simulink model "RASCAL72_cl"  (R2017b)
settings: Solver=FixedStepDiscrete  StartTime=0.0  StopTime=100  RelTol=1e-3  EnableMultiTasking=on
values from neighbouring files (symbols this model uses):
  CD0 = 0.0164    [Final_Project_START.m]
  CDa_200 = [0.53 0.53 0.53 0.53 0.53 0.53 0.53 0.53 0.53 0.53 0.53 0.53 ... (25 elements, 5x5)]    [C1o_200.mat]    (also in CDa_200.mat; CLadot_200.mat; CLde.mat; CLo_200.mat)
  CDde_200 = [0 0 0 0 0 0 0 0 0 0 0 0 ... (25 elements, 5x5)]    [C1o_200.mat]    (also in CDde_200.mat; CLadot_200.mat; CLde.mat; CLo_200.mat)
  CDq_200 = [0 0 0 0 0 0 0 0 0 0 0 0 ... (25 elements, 5x5)]    [C1o_200.mat]    (also in CDq_200.mat; CLadot_200.mat; CLde.mat; CLo_200.mat)
  CL0 = 0.21    [Final_Project_START.m]
  Cl0 = 0    [Final_Project_START.m]
  CLa_200 = [5.326215664 5.440234265 5.741037107 5.849899088 5.539928921 5.331372284 5.445390885 5.746766685 5.849899088 5.539355963 5.335955946 5.449401589 ... (25 elements, 5x5)]    [C1o_200.mat]    (also in CLa_200.mat; CLadot_200.mat; CLde.mat; CLo_200.mat)
  ClB_200 = [-0.052500123 -0.052614714 -0.052614714 -0.05294703 -0.053136106 -0.052523041 -0.052649092 -0.052666281 -0.053015785 -0.05322205 -0.052545959 -0.0525345 ... (25 elements, 5x5)]    [C1B_200.mat]    (also in C1o_200.mat; CLadot_200.mat; Cma_200.mat; Cmadot_200.mat)
  Clda_200 = [0.03678389 0.037299552 0.037299552 0.036726595 0.035580679 0.03678389 0.037299552 0.037299552 0.036726595 0.035580679 0.03678389 0.037299552 ... (25 elements, 5x5)]    [C1da_200.mat]    (also in C1o_200.mat = [0.000642 0.000651 0.000651 0.000641 0.000621 0.000642 0.000; CLadot_200.mat = [0.000642 0.000651 0.000651 0.000641 0.000621 0.000642 0.000; Cma_200.mat = [0.000642 0.000651 0.000651 0.000641 0.000621 0.000642 0.000; Cmadot_200.mat = [0.000642 0.000651 0.000651 0.000641 0.000621 0.000642 0.000)
  CLde_200 = [0.001609 0.00164 0.001639 0.001604 0.001542 0.001609 0.00164 0.001639 0.001604 0.001542 0.001609 0.00164 ... (25 elements, 5x5)]    [C1o_200.mat]    (also in CLadot_200.mat; CLde.mat; CLde_200.mat = [0.092188909 0.093965078 0.093907783 0.09190243 0.088350092 ; CLo_200.mat)
  Cldr_200 = [-5.72958e-05 0 5.72958e-05 0.000114592 0.000171887 -5.72958e-05 0 5.72958e-05 0.000114592 0.000171887 -5.72958e-05 0 ... (25 elements, 5x5)]    [C1dr_200.mat]    (also in C1o_200.mat = [-1e-06 0 1e-06 2e-06 3e-06 -1e-06 0 1e-06 2e-06 3e-06 -1e-0; CLadot_200.mat = [-1e-06 0 1e-06 2e-06 3e-06 -1e-06 0 1e-06 2e-06 3e-06 -1e-0; Cma_200.mat = [-1e-06 0 1e-06 2e-06 3e-06 -1e-06 0 1e-06 2e-06 3e-06 -1e-0; Cmadot_200.mat = [-1e-06 0 1e-06 2e-06 3e-06 -1e-06 0 1e-06 2e-06 3e-06 -1e-0)
  Clp_200 = [-0.448740545 -0.460829955 -0.490337281 -0.496124155 -0.462205053 -0.448740545 -0.460772659 -0.490279985 -0.496009563 -0.461861279 -0.448797841 -0.460829955 ... (25 elements, 5x5)]    [C1o_200.mat]    (also in C1p_200.mat; CLadot_200.mat; Cma_200.mat; Cmadot_200.mat)
  CLq_200 = [9.310564171 9.310564171 9.310564171 9.310564171 9.310564171 9.344941639 9.344941639 9.344941639 9.344941639 9.344941639 9.373589528 9.373589528 ... (25 elements, 5x5)]    [C1o_200.mat]    (also in CLadot_200.mat; CLde.mat; CLo_200.mat; CLq_200.mat)
  Clr_200 = [-0.074885584 0.016254813 0.110122488 0.213369483 0.308595068 -0.07494288 0.016260542 0.11023708 0.21354137 0.308824252 -0.075000175 0.016272001 ... (25 elements, 5x5)]    [C1o_200.mat]    (also in C1r_200.mat; CLadot_200.mat; CLde.mat; CLo_200.mat)
  Cm0 = 0    [Final_Project_START.m]
  Cma_200 = [-1.61689 -1.94061 -2.12224 -2.54508 -2.95302 -1.61918 -1.94978 -2.1314 -2.55367 -2.96506 -1.62319 -1.9578 ... (25 elements, 5x5)]    [C1o_200.mat]    (also in CLadot_200.mat; CLde.mat; CLo_200.mat; CLq_200.mat)
  Cmde_200 = [-0.002239 -0.002272 -0.00227 -0.00223 -0.002161 -0.002239 -0.002272 -0.00227 -0.00223 -0.002161 -0.002239 -0.002272 ... (25 elements, 5x5)]    [C1o_200.mat]    (also in CLadot_200.mat; CLde.mat; CLo_200.mat; CLq_200.mat)
  Cmq_200 = [-17.06841272 -17.06841272 -17.06841272 -17.06841272 -17.06841272 -17.17154512 -17.17154512 -17.17154512 -17.17154512 -17.17154512 -17.25175921 -17.25175921 ... (25 elements, 5x5)]    [C1o_200.mat]    (also in CLadot_200.mat; CLde.mat; CLo_200.mat; CLq_200.mat)
  Cn0 = 0    [Final_Project_START.m]
  CnB_200 = [0.029759428 0.029759428 0.029759428 0.029759428 0.029759428 0.028264008 0.028264008 0.028264008 0.028264008 0.028264008 0.027209766 0.027209766 ... (25 elements, 5x5)]    [C1o_200.mat]    (also in CLadot_200.mat; CLde.mat; CLo_200.mat; CLq_200.mat)
  Cnda_200 = [-4.5e-05 -2.9e-05 -1.1e-05 6e-06 2.2e-05 -4.5e-05 -2.9e-05 -1.1e-05 6e-06 2.2e-05 -4.5e-05 -2.9e-05 ... (25 elements, 5x5)]    [C1o_200.mat]    (also in CLadot_200.mat; CLde.mat; CLo_200.mat; CLq_200.mat)
  Cndr_200 = [0.000151 0.000159 0.000163 0.000164 0.00016 0.000151 0.000159 0.000163 0.000164 0.00016 0.000151 0.000159 ... (25 elements, 5x5)]    [C1o_200.mat]    (also in CLadot_200.mat; CLde.mat; CLo_200.mat; CLq_200.mat)
  Cnp_200 = [0.038193 0.000534 -0.03759 -0.07993 -0.12032 0.039712 0.000373 -0.03967 -0.08394 -0.12594 0.040583 0.00028 ... (25 elements, 5x5)]    [C1o_200.mat]    (also in CLadot_200.mat; CLde.mat; CLo_200.mat; CLq_200.mat)
  Cnr_200 = [-0.040473739 -0.043229666 -0.042771299 -0.038405361 -0.030859507 -0.040015372 -0.042908809 -0.042244178 -0.037247986 -0.028751022 -0.039728894 -0.042702544 ... (25 elements, 5x5)]    [C1o_200.mat]    (also in CLadot_200.mat; CLde.mat; CLo_200.mat; CLq_200.mat)
  CY0 = 0    [Final_Project_START.m]
  CYB_200 = [-0.504374747 -0.504374747 -0.504374747 -0.504374747 -0.504374747 -0.504374747 -0.504374747 -0.504374747 -0.504374747 -0.504374747 -0.504432043 -0.50432043 ... (25 elements, 5x5)]    [C1o_200.mat]    (also in CLadot_200.mat; CLde.mat; CLo_200.mat; CLq_200.mat)
  CYda_200 = [4e-06 2.7e-05 5e-05 7.1e-05 9.1e-05 4e-06 2.7e-05 5e-05 7.1e-05 9.1e-05 4e-06 2.7e-05 ... (25 elements, 5x5)]    [C1o_200.mat]    (also in CLadot_200.mat; CLde.mat; CLo_200.mat; CLq_200.mat)
  CYdr_200 = [-0.000731 -0.000766 -0.000782 -0.00078 -0.000759 -0.000731 -0.000766 -0.000782 -0.00078 -0.000759 -0.000731 -0.000766 ... (25 elements, 5x5)]    [C1o_200.mat]    (also in CLadot_200.mat; CLde.mat; CLo_200.mat; CLq_200.mat)
  CYp_200 = [-0.030521462 -0.058498991 -0.087204176 -0.119576292 -0.14919821 -0.029782346 -0.058613582 -0.088178205 -0.121581644 -0.152005703 -0.029358357 -0.058670878 ... (25 elements, 5x5)]    [C1o_200.mat]    (also in CLadot_200.mat; CLde.mat; CLo_200.mat; CLq_200.mat)
  CYr_200 = [0.026877 0.03248 0.035656 0.0363 0.03441 0.026877 0.03248 0.035656 0.0363 0.03441 0.026877 0.03248 ... (25 elements, 5x5)]    [C1o_200.mat]    (also in CLadot_200.mat; CLde.mat; CLo_200.mat; CLq_200.mat)
undefined symbols (not defined in the file or in its folder): airlib, B747, DiscIntNeverNeededParam, DT
(part 2 of 2)

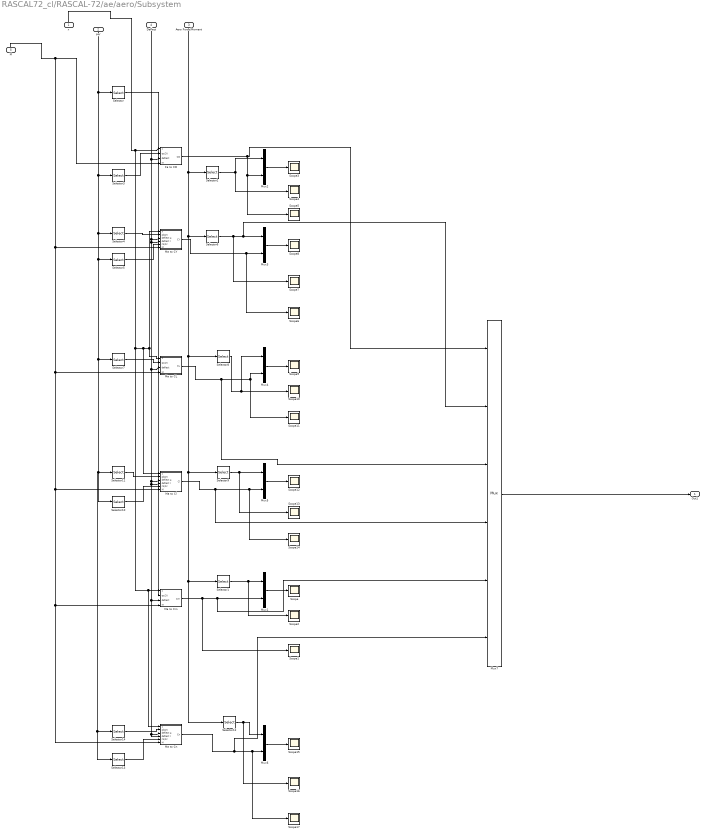
== system RASCAL72_cl/RASCAL-72/ae/aero/Subsystem ==
  x : Inport
  pqr : Inport  Port=2
  "Aero Force/Moment " : Inport  Port=3
  Deflect : Inport  Port=4
  M : Inport  Port=5
  Fa to CD : Subsystem
  Ma to CL : Subsystem
  Ma to CY : Subsystem
  Ma to Cl : Subsystem
  Ma to Cm : Subsystem
  Ma to Cn : Subsystem
  Mux{1..6} (6 alike) : Mux  Inputs=2
  Mux7 : Mux  Inputs=6
  Scope{,1..17} (18 alike) : Scope
  Selector : Selector  InputPortWidth=3  IndexOptions=Index vector (dialog)  Indices=2  OutputSizes=1
  Selector1 : Selector  InputPortWidth=6  IndexOptions=Index vector (dialog)  Indices=5  OutputSizes=1
  Selector10 : Selector  InputPortWidth=3  IndexOptions=Index vector (dialog)  Indices=3  OutputSizes=1
  Selector11 : Selector  InputPortWidth=3  IndexOptions=Index vector (dialog)  Indices=1  OutputSizes=1
  Selector12 : Selector  InputPortWidth=6  IndexOptions=Index vector (dialog)  Indices=6  OutputSizes=1
  Selector13 : Selector  InputPortWidth=3  IndexOptions=Index vector (dialog)  Indices=3  OutputSizes=1
  Selector14 : Selector  InputPortWidth=3  IndexOptions=Index vector (dialog)  Indices=1  OutputSizes=1
  Selector2 : Selector  InputPortWidth=6  IndexOptions=Index vector (dialog)  Indices=1  OutputSizes=1
  Selector3 : Selector  InputPortWidth=3  IndexOptions=Index vector (dialog)  Indices=2  OutputSizes=1
  Selector4 : Selector  InputPortWidth=3  IndexOptions=Index vector (dialog)  Indices=1  OutputSizes=1
  Selector5 : Selector  InputPortWidth=3  IndexOptions=Index vector (dialog)  Indices=3  OutputSizes=1
  Selector6 : Selector  InputPortWidth=6  IndexOptions=Index vector (dialog)  Indices=2  OutputSizes=1
  Selector7 : Selector  InputPortWidth=3  IndexOptions=Index vector (dialog)  Indices=2  OutputSizes=1
  Selector8 : Selector  InputPortWidth=6  IndexOptions=Index vector (dialog)  Indices=3  OutputSizes=1
  Selector9 : Selector  InputPortWidth=6  IndexOptions=Index vector (dialog)  Indices=4  OutputSizes=1
  Out1 : Outport
  wires:
  Selector14/1 -> Ma to Cn/2(pb/2V)
  Selector13/1 -> Ma to Cn/5(rb/2V)
  Selector6/1 -> Scope7/1, Mux7/2, Mux3/1
  Ma to CY/1(CY) -> Scope6/1, Mux3/2
  Mux2/1 -> Scope3/1
  Selector1/1 -> Scope2/1, Mux1/1
  Selector9/1 -> Scope13/1, Mux5/1
  pqr/1 -> Selector7/1, Selector10/1, Selector11/1, Selector14/1, Selector13/1, Selector5/1, Selector4/1, Selector3/1, Selector/1
  x/1 -> Fa to CD/1(x), Ma to Cl/1(x), Ma to CL/1(x), Ma to CY/1(x), Ma to Cn/1(x), Ma to Cm/1(x)
  "Aero Force/Moment "/1 -> Selector6/1, Selector8/1, Selector9/1, Selector12/1, Selector1/1, Selector2/1
  Ma to Cm/1(Cm) -> Scope1/1, Mux7/5, Mux1/2
  Selector3/1 -> Fa to CD/2(qc/2V)
  Selector/1 -> Ma to Cm/2(qc/2V)
  Mux3/1 -> Scope8/1
  Selector2/1 -> Scope4/1, Mux2/1
  Selector12/1 -> Scope16/1, Mux6/1
  Ma to Cn/1(Cn) -> Mux7/6, Scope17/1, Mux6/2
  Mux5/1 -> Scope12/1
  Selector5/1 -> Ma to CY/5(rb/2V)
  Selector7/1 -> Ma to CL/2(qc/2V)
  Mux4/1 -> Scope9/1
  Selector10/1 -> Ma to Cl/5(rb/2V)
  Selector11/1 -> Ma to Cl/2(pb/2V)
  Ma to Cl/1(Cl) -> Mux7/4, Scope14/1, Mux5/2
  Selector4/1 -> Ma to CY/2(pb/2V)
  Selector8/1 -> Scope10/1, Mux4/1
  Deflect/1 -> Fa to CD/3(deflect), Ma to CY/3(deflect a), Ma to CY/4(deflect r), Ma to CL/3(deflect), Ma to Cl/3(deflect a), Ma to Cm/3(deflect), Ma to Cn/3(deflect a), Ma to Cn/4(deflect r), Ma to Cl/4(deflect r)
  Mux1/1 -> Scope/1
  Mux6/1 -> Scope15/1
  M/1 -> Fa to CD/4(M), Ma to CY/6(M), Ma to Cl/6(M), Ma to Cm/4(M), Ma to Cn/6(M), Ma to CL/4("M ")
  Fa to CD/1(CD) -> Mux7/1, Scope5/1, Mux2/2
  Ma to CL/1(CL) -> Mux7/3, Mux4/2, Scope11/1
  Mux7/1 -> Out1/1

== system RASCAL72_cl/RASCAL-72/ae/dl/0 ==

== system RASCAL72_cl/RASCAL-72/ae/fmdims/0 ==

== system RASCAL72_cl/RASCAL-72/eqm/ODE/0 ==

== system RASCAL72_cl/RASCAL-72/eqm/ODE/Eulerdot ==
  note: yeul=[psi dot; theta dot; phi dot]
  note: ueul=[x;Ftot;Mtot;yhlp]
  ueul : Inport
  0 : Subsystem
      mask Display: disp('EULERDOT\nM.O. Rauw, October 1997')
  Mux1 : Mux  Inputs=[29 1]
  Mux2 : Mux  Inputs=3
  phi dot : Fcn  Expr=u[4] + u[30]*u[26]
  psi dot : Fcn  Expr=(u[5]*u[28] + u[6]*u[29])/u[27]
  theta dot : Fcn  Expr=u[5]*u[29] - u[6]*u[28]
  yeul : Outport
  wires:
  Mux1/1 -> phi dot/1
  phi dot/1 -> Mux2/3
  Mux2/1 -> yeul/1
  theta dot/1 -> Mux2/2
  psi dot/1 -> Mux1/2, Mux2/1
  ueul/1 -> psi dot/1, Mux1/1, theta dot/1

== system RASCAL72_cl/RASCAL-72/eqm/ODE/Vabdot ==
  note: uVab=[x;Ftot;Mtot;yhlp]
  note: yVab=[V dot;alpha dot;beta dot]
  uVab : Inport
  0 : Subsystem
      mask Display: disp('VABDOT\nM.O. Rauw, October 1997')
  Mux2 : Mux  Inputs=3
  V dot : Fcn  Expr=(u[13]*u[19]*u[21]+u[14]*u[22]+u[15]*u[20]*u[21])/m
  alpha dot : Fcn  Expr=(-u[13]*u[20]+u[15]*u[19])/(m*u[1]*u[21]) - u[23]*(u[4]*u[19]+u[6]*u[20]) + u[5]
  beta dot : Fcn  Expr=(-u[13]*u[19]*u[22]+u[14]*u[21]-u[15]*u[20]*u[22])/(m*u[1]) + u[4]*u[20] - u[6]*u[19]
  yVab : Outport
  wires:
  Mux2/1 -> yVab/1
  uVab/1 -> V dot/1, beta dot/1, alpha dot/1
  alpha dot/1 -> Mux2/2
  V dot/1 -> Mux2/1
  beta dot/1 -> Mux2/3

== system RASCAL72_cl/RASCAL-72/eqm/ODE/pqrdot ==
  note: [p q r]'
  note: [L M N]'
  note: Here: ypqr = GM2*ytmp
  note: ytmp
  note: ypqr=[p dot;q dot;r dot]
  note: upqr=[x;Ftot;Mtot;yhlp]
  note: ytmp = [L; M; N; p^2; pq; pr; q^2; qr; r^2]
  upqr : Inport
  0 : Subsystem
      mask Display: disp('PQRDOT\nM.O. Rauw, October 1997')
  Demux : Demux  Outputs=[3 3 9 3 11]
  Fcn : Fcn  Expr=u[1]^2
  Fcn1 : Fcn  Expr=u[1]*u[2]
  Fcn2 : Fcn  Expr=u[1]*u[3]
  Fcn3 : Fcn  Expr=u[2]^2
  Fcn4 : Fcn  Expr=u[2]*u[3]
  Fcn5 : Fcn  Expr=u[3]^2
  "GM2 " : Subsystem  mask(State Space){M=GM2}
      mask prompts: M "Matrix"
      mask Display: disp('Matrix\nGain')
  Mux : Mux  Inputs=[3 1 1 1 1 1 1]
  Terminator1 : Terminator
  Terminator2 : Terminator
  Terminator3 : Terminator
  ypqr : Outport
  wires:
  upqr/1 -> Demux/1
  Demux/1 -> Terminator3/1
  Demux/5 -> Terminator2/1
  Demux/3 -> Terminator1/1
  Demux/2 -> Fcn1/1, Fcn/1, Fcn2/1, Fcn4/1, Fcn5/1, Fcn3/1
  Demux/4 -> Mux/1
  Fcn/1 -> Mux/2
  Fcn1/1 -> Mux/3
  Fcn2/1 -> Mux/4
  Fcn3/1 -> Mux/5
  Fcn4/1 -> Mux/6
  Fcn5/1 -> Mux/7
  "GM2 "/1(Out1) -> ypqr/1
  Mux/1 -> "GM2 "/1(In1)

== system RASCAL72_cl/RASCAL-72/eqm/ODE/xyHdot ==
  note: yxyH=[xe dot; ye dot; H dot]
  note: uxyH=[x;Ftot;Mtot;yhlp]
  ybvel* : Inport
  uxYH : Inport  Port=2
  0 : Subsystem
      mask Display: disp('XYHDOT\nM.O. Rauw, October 1997')
  H dot : Fcn  Expr=u[30]*u[26] - (u[31]*u[28]+u[32]*u[29])*u[27]
  Mux2 : Mux  Inputs=[29 3]
  Mux3 : Mux  Inputs=2
  Mux4 : Mux  Inputs=[29 2]
  Mux5 : Mux  Inputs=3
  tmp1 : Fcn  Expr=u[30]*u[27] + (u[31]*u[28]+u[32]*u[29])*u[26]
  tmp2 : Fcn  Expr=u[31]*u[29] - u[32]*u[28]
  xe dot : Fcn  Expr=u[30]*u[25] - u[31]*u[24]
  ye dot : Fcn  Expr=u[30]*u[24] + u[31]*u[25]
  yxyH : Outport
  wires:
  tmp1/1 -> Mux3/1
  H dot/1 -> Mux5/3
  xe dot/1 -> Mux5/1
  tmp2/1 -> Mux3/2
  ye dot/1 -> Mux5/2
  Mux5/1 -> yxyH/1
  Mux4/1 -> ye dot/1, xe dot/1
  Mux2/1 -> H dot/1, tmp2/1, tmp1/1
  Mux3/1 -> Mux4/2
  ybvel*/1 -> Mux2/2
  uxYH/1 -> Mux4/1, Mux2/1

== system RASCAL72_cl/RASCAL-72/eqm/uvw/0 ==

== system RASCAL72_cl/RASCAL-72/eqm/xdotcorr/0 ==

== system RASCAL72_cl/RASCAL-72/out/accel/0 ==

== system RASCAL72_cl/RASCAL-72/out/fp/0 ==

== system RASCAL72_cl/RASCAL-72/out/uvwdot/0 ==

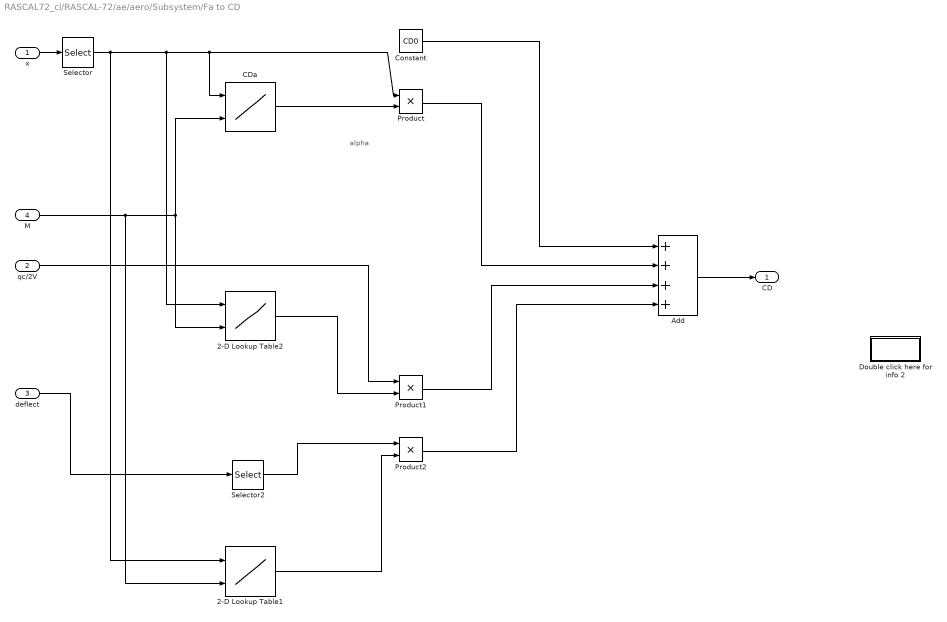
== system RASCAL72_cl/RASCAL-72/ae/aero/Subsystem/Fa to CD ==
  note: alpha
  x : Inport
  qc/2V : Inport  Port=2
  deflect : Inport  Port=3
  M : Inport  Port=4
  2-D Lookup Table1 : Lookup_n-D  BreakpointsForDimension1=[-10 -5 0 5 10]  BreakpointsForDimension2=[0.0294 0.04408 0.05877 0.07347 0.08816]  Table=CDde_200  InternalRulePriority=Speed  RndMeth=Simplest  InputSameDT=on
  2-D Lookup Table2 : Lookup_n-D  BreakpointsForDimension1=[-10 -5 0 5 10]  BreakpointsForDimension2=[0.0294 0.04408 0.05877 0.07347 0.08816]  Table=CDq_200  InternalRulePriority=Speed  RndMeth=Simplest  InputSameDT=on
  Add : Sum  Inputs=++++
  CDa : Lookup_n-D  BreakpointsForDimension1=[-10 -5 0 5 10]  BreakpointsForDimension2=[0.0294 0.04408 0.05877 0.07347 0.08816]  Table=CDa_200  InternalRulePriority=Speed  RndMeth=Simplest  InputSameDT=on
  Constant : Constant  Value=CD0
  Double click here for info 2 : Subsystem
      mask Display: disp('Output\nSignals')
  Product : Product
  Product1 : Product
  Product2 : Product
  Selector : Selector  InputPortWidth=12  IndexOptions=Index vector (dialog)  Indices=2  OutputSizes=1
  Selector2 : Selector  InputPortWidth=4  IndexOptions=Index vector (dialog)  Indices=1  OutputSizes=1
  CD : Outport
  wires:
  deflect/1 -> Selector2/1
  Product1/1 -> Add/3
  Product2/1 -> Add/4
  2-D Lookup Table1/1 -> Product2/2
  Selector2/1 -> Product2/1
  2-D Lookup Table2/1 -> Product1/2
  qc/2V/1 -> Product1/1
  Product/1 -> Add/2
  CDa/1 -> Product/2
  x/1 -> Selector/1
  Add/1 -> CD/1
  Constant/1 -> Add/1
  M/1 -> 2-D Lookup Table1/2, 2-D Lookup Table2/2, CDa/2
  Selector/1 -> 2-D Lookup Table2/1, CDa/1, Product/1, 2-D Lookup Table1/1

== system RASCAL72_cl/RASCAL-72/ae/aero/Subsystem/Ma to CL ==
  note: alpha
  x : Inport
  qc/2V : Inport  Port=2
  deflect : Inport  Port=3
  "M " : Inport  Port=4
  2-D Lookup Table : Lookup_n-D  BreakpointsForDimension1=[-10 -5 0 5 10]  BreakpointsForDimension2=[0.0294 0.04408 0.05877 0.07347 0.08816]  Table=CLa_200  InternalRulePriority=Speed  RndMeth=Simplest  InputSameDT=on
  2-D Lookup Table1 : Lookup_n-D  BreakpointsForDimension1=[-10 -5 0 5 10]  BreakpointsForDimension2=[0.0294 0.04408 0.05877 0.07347 0.08816]  Table=CLq_200  InternalRulePriority=Speed  RndMeth=Simplest  InputSameDT=on
  2-D Lookup Table2 : Lookup_n-D  BreakpointsForDimension1=[-10 -5 0 5 10]  BreakpointsForDimension2=[0.0294 0.04408 0.05877 0.07347 0.08816]  Table=CLde_200  InternalRulePriority=Speed  RndMeth=Simplest  InputSameDT=on
  Add : Sum  Inputs=++++
  Constant : Constant  Value=CL0
  Double click here for info 2 : Subsystem
      mask Display: disp('Output\nSignals')
  Product : Product
  Product1 : Product
  Product2 : Product
  Selector : Selector  InputPortWidth=12  IndexOptions=Index vector (dialog)  Indices=2  OutputSizes=1
  Selector2 : Selector  InputPortWidth=4  IndexOptions=Index vector (dialog)  Indices=1  OutputSizes=1
  CL : Outport
  wires:
  Constant/1 -> Add/1
  Add/1 -> CL/1
  x/1 -> Selector/1
  Selector/1 -> 2-D Lookup Table/1, 2-D Lookup Table2/1, 2-D Lookup Table1/1, Product/1
  2-D Lookup Table/1 -> Product/2
  Product/1 -> Add/2
  qc/2V/1 -> Product1/1
  2-D Lookup Table1/1 -> Product1/2
  Selector2/1 -> Product2/1
  2-D Lookup Table2/1 -> Product2/2
  Product2/1 -> Add/4
  Product1/1 -> Add/3
  deflect/1 -> Selector2/1
  "M "/1 -> 2-D Lookup Table2/2, 2-D Lookup Table1/2, 2-D Lookup Table/2

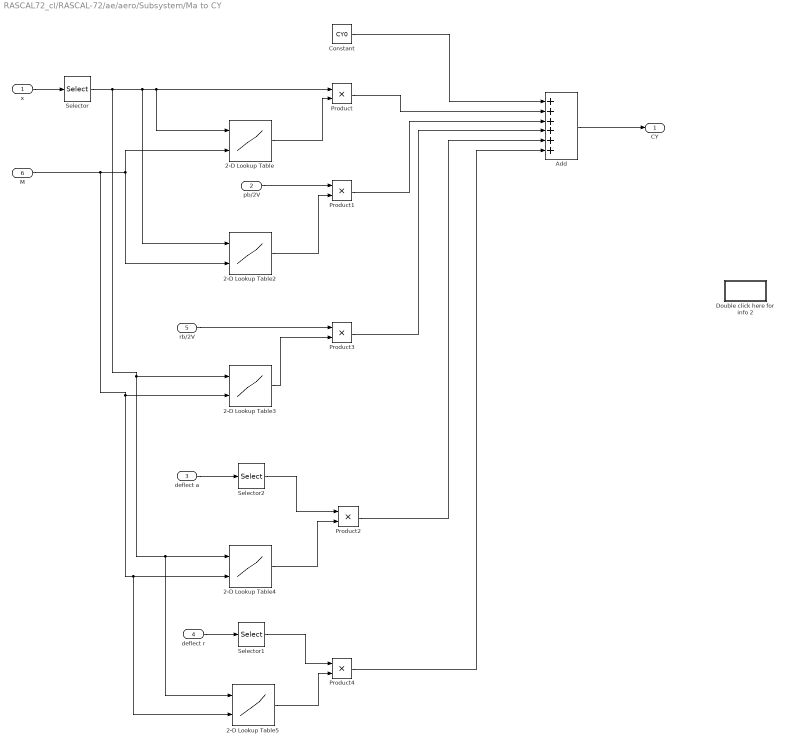
== system RASCAL72_cl/RASCAL-72/ae/aero/Subsystem/Ma to CY ==
  x : Inport
  pb/2V : Inport  Port=2
  deflect a : Inport  Port=3
  deflect r : Inport  Port=4
  rb/2V : Inport  Port=5
  M : Inport  Port=6
  2-D Lookup Table : Lookup_n-D  BreakpointsForDimension1=[-10 -5 0 5 10]  BreakpointsForDimension2=[0.0294 0.04408 0.05877 0.07347 0.08816]  Table=CYB_200  InternalRulePriority=Speed  RndMeth=Simplest  InputSameDT=on
  2-D Lookup Table2 : Lookup_n-D  BreakpointsForDimension1=[-10 -5 0 5 10]  BreakpointsForDimension2=[0.0294 0.04408 0.05877 0.07347 0.08816]  Table=CYp_200  InternalRulePriority=Speed  RndMeth=Simplest  InputSameDT=on
  2-D Lookup Table3 : Lookup_n-D  BreakpointsForDimension1=[-10 -5 0 5 10]  BreakpointsForDimension2=[0.0294 0.04408 0.05877 0.07347 0.08816]  Table=CYr_200  InternalRulePriority=Speed  RndMeth=Simplest  InputSameDT=on
  2-D Lookup Table4 : Lookup_n-D  BreakpointsForDimension1=[-10 -5 0 5 10]  BreakpointsForDimension2=[0.0294 0.04408 0.05877 0.07347 0.08816]  Table=CYda_200  InternalRulePriority=Speed  RndMeth=Simplest  InputSameDT=on
  2-D Lookup Table5 : Lookup_n-D  BreakpointsForDimension1=[-10 -5 0 5 10]  BreakpointsForDimension2=[0.0294 0.04408 0.05877 0.07347 0.08816]  Table=CYdr_200  InternalRulePriority=Speed  RndMeth=Simplest  InputSameDT=on
  Add : Sum  Inputs=++++++
  Constant : Constant  Value=CY0
  Double click here for info 2 : Subsystem
      mask Display: disp('Output\nSignals')
  Product{,1..4} (5 alike) : Product
  Selector : Selector  InputPortWidth=12  IndexOptions=Index vector (dialog)  Indices=2  OutputSizes=1
  Selector1 : Selector  InputPortWidth=4  IndexOptions=Index vector (dialog)  Indices=3  OutputSizes=1
  Selector2 : Selector  InputPortWidth=4  IndexOptions=Index vector (dialog)  Indices=2  OutputSizes=1
  CY : Outport
  wires:
  Constant/1 -> Add/1
  Add/1 -> CY/1
  x/1 -> Selector/1
  Selector/1 -> 2-D Lookup Table2/1, 2-D Lookup Table/1, Product/1, 2-D Lookup Table5/1, 2-D Lookup Table4/1, 2-D Lookup Table3/1
  2-D Lookup Table/1 -> Product/2
  Product/1 -> Add/2
  pb/2V/1 -> Product1/1
  2-D Lookup Table2/1 -> Product1/2
  Selector2/1 -> Product2/1
  2-D Lookup Table4/1 -> Product2/2
  Product1/1 -> Add/3
  deflect a/1 -> Selector2/1
  Selector1/1 -> Product4/1
  2-D Lookup Table5/1 -> Product4/2
  Product4/1 -> Add/6
  2-D Lookup Table3/1 -> Product3/2
  Product3/1 -> Add/4
  Product2/1 -> Add/5
  deflect r/1 -> Selector1/1
  rb/2V/1 -> Product3/1
  M/1 -> 2-D Lookup Table5/2, 2-D Lookup Table4/2, 2-D Lookup Table3/2, 2-D Lookup Table2/2, 2-D Lookup Table/2

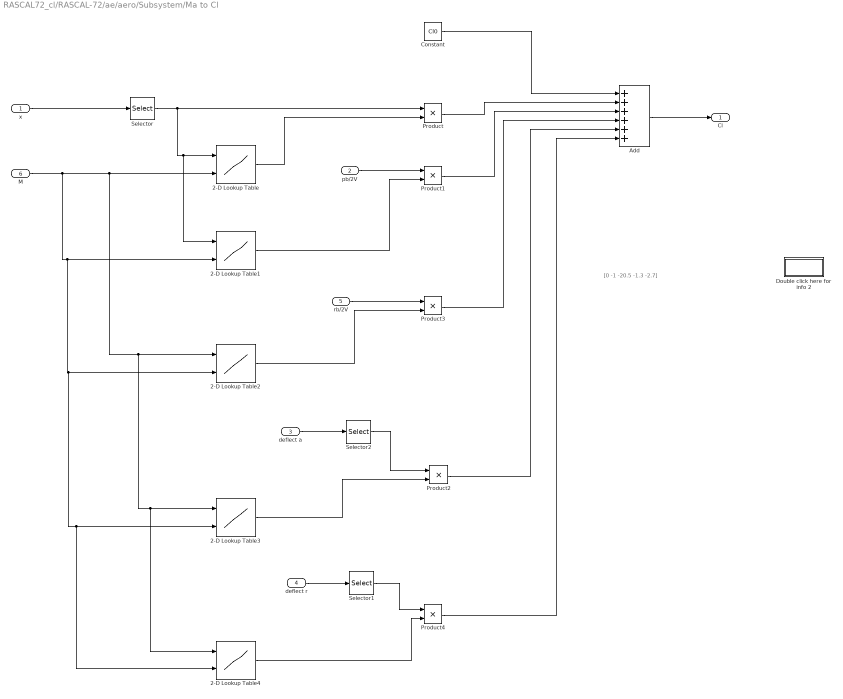
== system RASCAL72_cl/RASCAL-72/ae/aero/Subsystem/Ma to Cl ==
  note: [0 -1 -20.5 -1.3 -2.7]
  x : Inport
  pb/2V : Inport  Port=2
  deflect a : Inport  Port=3
  deflect r : Inport  Port=4
  rb/2V : Inport  Port=5
  M : Inport  Port=6
  2-D Lookup Table : Lookup_n-D  BreakpointsForDimension1=[-10 -5 0 5 10]  BreakpointsForDimension2=[0.0294 0.04408 0.05877 0.07347 0.08816]  Table=ClB_200  InternalRulePriority=Speed  RndMeth=Simplest  InputSameDT=on
  2-D Lookup Table1 : Lookup_n-D  BreakpointsForDimension1=[-10 -5 0 5 10]  BreakpointsForDimension2=[0.0294 0.04408 0.05877 0.07347 0.08816]  Table=Clp_200  InternalRulePriority=Speed  RndMeth=Simplest  InputSameDT=on
  2-D Lookup Table2 : Lookup_n-D  BreakpointsForDimension1=[-10 -5 0 5 10]  BreakpointsForDimension2=[0.0294 0.04408 0.05877 0.07347 0.08816]  Table=Clr_200  InternalRulePriority=Speed  RndMeth=Simplest  InputSameDT=on
  2-D Lookup Table3 : Lookup_n-D  BreakpointsForDimension1=[-10 -5 0 5 10]  BreakpointsForDimension2=[0.0294 0.04408 0.05877 0.07347 0.08816]  Table=Clda_200  InternalRulePriority=Speed  RndMeth=Simplest  InputSameDT=on
  2-D Lookup Table4 : Lookup_n-D  BreakpointsForDimension1=[-10 -5 0 5 10]  BreakpointsForDimension2=[0.0294 0.04408 0.05877 0.07347 0.08816]  Table=Cldr_200  InternalRulePriority=Speed  RndMeth=Simplest  InputSameDT=on
  Add : Sum  Inputs=++++++
  Constant : Constant  Value=Cl0
  Double click here for info 2 : Subsystem
      mask Display: disp('Output\nSignals')
  Product{,1..4} (5 alike) : Product
  Selector : Selector  InputPortWidth=12  IndexOptions=Index vector (dialog)  Indices=2  OutputSizes=1
  Selector1 : Selector  InputPortWidth=4  IndexOptions=Index vector (dialog)  Indices=3  OutputSizes=1
  Selector2 : Selector  InputPortWidth=4  IndexOptions=Index vector (dialog)  Indices=2  OutputSizes=1
  Cl : Outport
  wires:
  rb/2V/1 -> Product3/1
  deflect r/1 -> Selector1/1
  Product2/1 -> Add/5
  Product3/1 -> Add/4
  2-D Lookup Table2/1 -> Product3/2
  Product4/1 -> Add/6
  2-D Lookup Table4/1 -> Product4/2
  Selector1/1 -> Product4/1
  deflect a/1 -> Selector2/1
  Product1/1 -> Add/3
  2-D Lookup Table3/1 -> Product2/2
  Selector2/1 -> Product2/1
  2-D Lookup Table1/1 -> Product1/2
  pb/2V/1 -> Product1/1
  Product/1 -> Add/2
  2-D Lookup Table/1 -> Product/2
  Selector/1 -> 2-D Lookup Table1/1, 2-D Lookup Table/1, Product/1
  x/1 -> Selector/1
  Add/1 -> Cl/1
  Constant/1 -> Add/1
  M/1 -> 2-D Lookup Table4/2, 2-D Lookup Table3/2, 2-D Lookup Table2/2, 2-D Lookup Table1/2, 2-D Lookup Table4/1, 2-D Lookup Table3/1, 2-D Lookup Table2/1, 2-D Lookup Table/2

== system RASCAL72_cl/RASCAL-72/ae/aero/Subsystem/Ma to Cm ==
  note: alpha
  x : Inport
  qc/2V : Inport  Port=2
  deflect : Inport  Port=3
  M : Inport  Port=4
  2-D Lookup Table : Lookup_n-D  BreakpointsForDimension1=[-10 -5 0 5 10]  BreakpointsForDimension2=[0.0294 0.04408 0.05877 0.07347 0.08816]  Table=Cma_200  InternalRulePriority=Speed  RndMeth=Simplest  InputSameDT=on
  2-D Lookup Table1 : Lookup_n-D  BreakpointsForDimension1=[-10 -5 0 5 10]  BreakpointsForDimension2=[0.0294 0.04408 0.05877 0.07347 0.08816]  Table=Cmde_200  InternalRulePriority=Speed  RndMeth=Simplest  InputSameDT=on
  2-D Lookup Table2 : Lookup_n-D  BreakpointsForDimension1=[-10 -5 0 5 10]  BreakpointsForDimension2=[0.0294 0.04408 0.05877 0.07347 0.08816]  Table=Cmq_200  InternalRulePriority=Speed  RndMeth=Simplest  InputSameDT=on
  Add : Sum  Inputs=++++  RndMeth=Nearest
  Constant : Constant  Value=Cm0
  Double click here for info 2 : Subsystem
      mask Display: disp('Output\nSignals')
  Product : Product
  Product1 : Product
  Product2 : Product
  Selector : Selector  InputPortWidth=12  IndexOptions=Index vector (dialog)  Indices=2  OutputSizes=1
  Selector2 : Selector  InputPortWidth=4  IndexOptions=Index vector (dialog)  Indices=1  OutputSizes=1
  Cm : Outport
  wires:
  Constant/1 -> Add/1
  Add/1 -> Cm/1
  x/1 -> Selector/1
  Product/1 -> Add/2
  qc/2V/1 -> Product1/1
  Selector2/1 -> Product2/1
  Product2/1 -> Add/4
  Product1/1 -> Add/3
  deflect/1 -> Selector2/1
  M/1 -> 2-D Lookup Table/2, 2-D Lookup Table1/2, 2-D Lookup Table2/2
  2-D Lookup Table/1 -> Product/2
  2-D Lookup Table2/1 -> Product1/2
  Selector/1 -> 2-D Lookup Table/1, 2-D Lookup Table2/1, 2-D Lookup Table1/1, Product/1
  2-D Lookup Table1/1 -> Product2/2

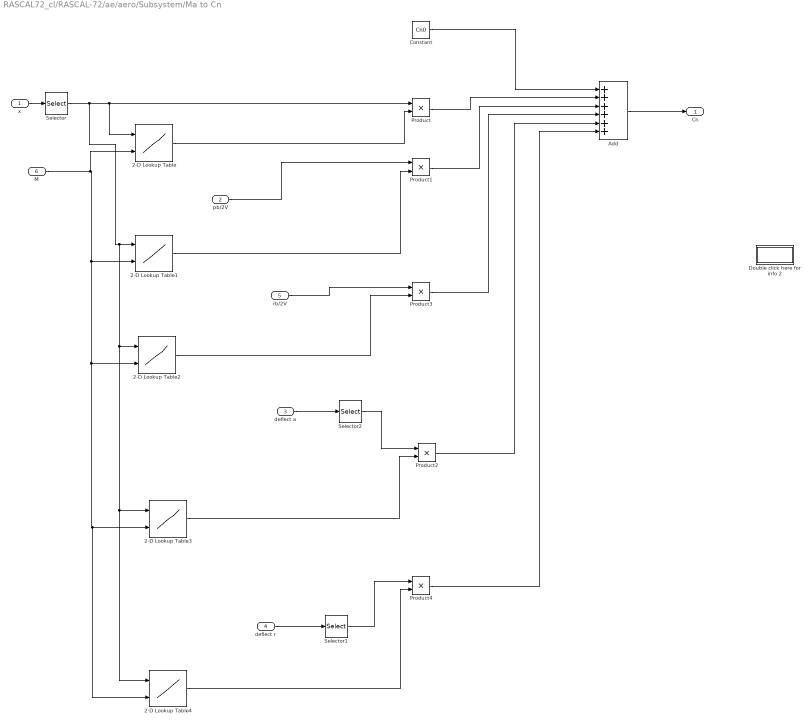
== system RASCAL72_cl/RASCAL-72/ae/aero/Subsystem/Ma to Cn ==
  x : Inport
  pb/2V : Inport  Port=2
  deflect a : Inport  Port=3
  deflect r : Inport  Port=4
  rb/2V : Inport  Port=5
  M : Inport  Port=6
  2-D Lookup Table : Lookup_n-D  BreakpointsForDimension1=[-10 -5 0 5 10]  BreakpointsForDimension2=[0.0294 0.04408 0.05877 0.07347 0.08816]  Table=CnB_200  InternalRulePriority=Speed  RndMeth=Simplest  InputSameDT=on
  2-D Lookup Table1 : Lookup_n-D  BreakpointsForDimension1=[-10 -5 0 5 10]  BreakpointsForDimension2=[0.0294 0.04408 0.05877 0.07347 0.08816]  Table=Cnp_200  InternalRulePriority=Speed  RndMeth=Simplest  InputSameDT=on
  2-D Lookup Table2 : Lookup_n-D  BreakpointsForDimension1=[-10 -5 0 5 10]  BreakpointsForDimension2=[0.0294 0.04408 0.05877 0.07347 0.08816]  Table=Cnr_200  InternalRulePriority=Speed  RndMeth=Simplest  InputSameDT=on
  2-D Lookup Table3 : Lookup_n-D  BreakpointsForDimension1=[-10 -5 0 5 10]  BreakpointsForDimension2=[0.0294 0.04408 0.05877 0.07347 0.08816]  Table=Cnda_200  InternalRulePriority=Speed  RndMeth=Simplest  InputSameDT=on
  2-D Lookup Table4 : Lookup_n-D  BreakpointsForDimension1=[-10 -5 0 5 10]  BreakpointsForDimension2=[0.0294 0.04408 0.05877 0.07347 0.08816]  Table=Cndr_200  InternalRulePriority=Speed  RndMeth=Simplest  InputSameDT=on
  Add : Sum  Inputs=++++++
  Constant : Constant  Value=Cn0
  Double click here for info 2 : Subsystem
      mask Display: disp('Output\nSignals')
  Product{,1..4} (5 alike) : Product
  Selector : Selector  InputPortWidth=12  IndexOptions=Index vector (dialog)  Indices=2  OutputSizes=1
  Selector1 : Selector  InputPortWidth=4  IndexOptions=Index vector (dialog)  Indices=3  OutputSizes=1
  Selector2 : Selector  InputPortWidth=4  IndexOptions=Index vector (dialog)  Indices=2  OutputSizes=1
  Cn : Outport
  wires:
  Constant/1 -> Add/1
  Add/1 -> Cn/1
  x/1 -> Selector/1
  Selector/1 -> 2-D Lookup Table2/1, 2-D Lookup Table3/1, 2-D Lookup Table4/1, 2-D Lookup Table1/1, 2-D Lookup Table/1, Product/1
  2-D Lookup Table/1 -> Product/2
  Product/1 -> Add/2
  pb/2V/1 -> Product1/1
  2-D Lookup Table1/1 -> Product1/2
  Selector2/1 -> Product2/1
  2-D Lookup Table3/1 -> Product2/2
  Product1/1 -> Add/3
  deflect a/1 -> Selector2/1
  Selector1/1 -> Product4/1
  2-D Lookup Table4/1 -> Product4/2
  Product4/1 -> Add/6
  2-D Lookup Table2/1 -> Product3/2
  Product3/1 -> Add/4
  Product2/1 -> Add/5
  deflect r/1 -> Selector1/1
  rb/2V/1 -> Product3/1
  M/1 -> 2-D Lookup Table4/2, 2-D Lookup Table3/2, 2-D Lookup Table2/2, 2-D Lookup Table1/2, 2-D Lookup Table/2

== system RASCAL72_cl/RASCAL-72/eqm/ODE/Eulerdot/0 ==

== system RASCAL72_cl/RASCAL-72/eqm/ODE/Vabdot/0 ==

== system RASCAL72_cl/RASCAL-72/eqm/ODE/pqrdot/0 ==

== system RASCAL72_cl/RASCAL-72/eqm/ODE/pqrdot/GM2  ==
  In1 : Inport
  Matrix Gain : StateSpace  A=[]  B=[]  C=[]  D=M  InitialCondition=0
  Out1 : Outport
  wires:
  Matrix Gain/1 -> Out1/1
  In1/1 -> Matrix Gain/1

== system RASCAL72_cl/RASCAL-72/eqm/ODE/xyHdot/0 ==

== system RASCAL72_cl/RASCAL-72/ae/aero/Subsystem/Fa to CD/Double click here for info 2 ==
  note: 01 v (m/s)
      | 02 alpha (rad)
      | 03 beta (rad)
      | 04 p (rad/s)
      | 05 q (rad/s)
      | 06 r  (rad/s)
      | 07 psi (rad)
      | 08 theta (rad)
      | 09 phi (rad)
      | 10 xe (m)
      | 11 ye (m)
      | 12 ze (m)
      | 13 v dot (m/s2)
      | 14 alpha dot (rad/s)
      | 15 beta dot (rad/s)
      | 16 p dot (rad/s2)
      | 17 q dot (rad/s2)
      | 18 r dot (rad/s2)
      | 19 fi dot (rad/s)
      | 20 theta dot (rad/s)
      | 21 psi dot (rad/s)
      | 22 xe dot (m/s)
      | 23 ye dot (m/s)
      | 24 ze dot (m/s)
      | 25 u dot (m/s2)
      | 26 v dot (m/s2)
      | 27 w dot (m/s2)
      | 28 pb/2v (rad)
      | 29 qc/v (rad)
      | 30 rb/v (rad)
      | 31 Ax (g)
      | 32 Ay (g)
      | 33 Az (g)
      | 34 ax (g)
      | 35 ay (g)
      | 36 az (g)
      | 37 delta elevators (rad)
      | 38 delta ailerons (rad)
      | 39 delta rudder (rad)
      | 40 delta stabs (rad)

== system RASCAL72_cl/RASCAL-72/ae/aero/Subsystem/Ma to CL/Double click here for info 2 ==
  note: 01 v (m/s)
      | 02 alpha (rad)
      | 03 beta (rad)
      | 04 p (rad/s)
      | 05 q (rad/s)
      | 06 r  (rad/s)
      | 07 psi (rad)
      | 08 theta (rad)
      | 09 phi (rad)
      | 10 xe (m)
      | 11 ye (m)
      | 12 ze (m)
      | 13 v dot (m/s2)
      | 14 alpha dot (rad/s)
      | 15 beta dot (rad/s)
      | 16 p dot (rad/s2)
      | 17 q dot (rad/s2)
      | 18 r dot (rad/s2)
      | 19 fi dot (rad/s)
      | 20 theta dot (rad/s)
      | 21 psi dot (rad/s)
      | 22 xe dot (m/s)
      | 23 ye dot (m/s)
      | 24 ze dot (m/s)
      | 25 u dot (m/s2)
      | 26 v dot (m/s2)
      | 27 w dot (m/s2)
      | 28 pb/2v (rad)
      | 29 qc/v (rad)
      | 30 rb/v (rad)
      | 31 Ax (g)
      | 32 Ay (g)
      | 33 Az (g)
      | 34 ax (g)
      | 35 ay (g)
      | 36 az (g)
      | 37 delta elevators (rad)
      | 38 delta ailerons (rad)
      | 39 delta rudder (rad)
      | 40 delta stabs (rad)

== system RASCAL72_cl/RASCAL-72/ae/aero/Subsystem/Ma to CY/Double click here for info 2 ==
  note: 01 v (m/s)
      | 02 alpha (rad)
      | 03 beta (rad)
      | 04 p (rad/s)
      | 05 q (rad/s)
      | 06 r  (rad/s)
      | 07 psi (rad)
      | 08 theta (rad)
      | 09 phi (rad)
      | 10 xe (m)
      | 11 ye (m)
      | 12 ze (m)
      | 13 v dot (m/s2)
      | 14 alpha dot (rad/s)
      | 15 beta dot (rad/s)
      | 16 p dot (rad/s2)
      | 17 q dot (rad/s2)
      | 18 r dot (rad/s2)
      | 19 fi dot (rad/s)
      | 20 theta dot (rad/s)
      | 21 psi dot (rad/s)
      | 22 xe dot (m/s)
      | 23 ye dot (m/s)
      | 24 ze dot (m/s)
      | 25 u dot (m/s2)
      | 26 v dot (m/s2)
      | 27 w dot (m/s2)
      | 28 pb/2v (rad)
      | 29 qc/v (rad)
      | 30 rb/v (rad)
      | 31 Ax (g)
      | 32 Ay (g)
      | 33 Az (g)
      | 34 ax (g)
      | 35 ay (g)
      | 36 az (g)
      | 37 delta elevators (rad)
      | 38 delta ailerons (rad)
      | 39 delta rudder (rad)
      | 40 delta stabs (rad)

== system RASCAL72_cl/RASCAL-72/ae/aero/Subsystem/Ma to Cl/Double click here for info 2 ==
  note: 01 v (m/s)
      | 02 alpha (rad)
      | 03 beta (rad)
      | 04 p (rad/s)
      | 05 q (rad/s)
      | 06 r  (rad/s)
      | 07 psi (rad)
      | 08 theta (rad)
      | 09 phi (rad)
      | 10 xe (m)
      | 11 ye (m)
      | 12 ze (m)
      | 13 v dot (m/s2)
      | 14 alpha dot (rad/s)
      | 15 beta dot (rad/s)
      | 16 p dot (rad/s2)
      | 17 q dot (rad/s2)
      | 18 r dot (rad/s2)
      | 19 fi dot (rad/s)
      | 20 theta dot (rad/s)
      | 21 psi dot (rad/s)
      | 22 xe dot (m/s)
      | 23 ye dot (m/s)
      | 24 ze dot (m/s)
      | 25 u dot (m/s2)
      | 26 v dot (m/s2)
      | 27 w dot (m/s2)
      | 28 pb/2v (rad)
      | 29 qc/v (rad)
      | 30 rb/v (rad)
      | 31 Ax (g)
      | 32 Ay (g)
      | 33 Az (g)
      | 34 ax (g)
      | 35 ay (g)
      | 36 az (g)
      | 37 delta elevators (rad)
      | 38 delta ailerons (rad)
      | 39 delta rudder (rad)
      | 40 delta stabs (rad)

== system RASCAL72_cl/RASCAL-72/ae/aero/Subsystem/Ma to Cm/Double click here for info 2 ==
  note: 01 v (m/s)
      | 02 alpha (rad)
      | 03 beta (rad)
      | 04 p (rad/s)
      | 05 q (rad/s)
      | 06 r  (rad/s)
      | 07 psi (rad)
      | 08 theta (rad)
      | 09 phi (rad)
      | 10 xe (m)
      | 11 ye (m)
      | 12 ze (m)
      | 13 v dot (m/s2)
      | 14 alpha dot (rad/s)
      | 15 beta dot (rad/s)
      | 16 p dot (rad/s2)
      | 17 q dot (rad/s2)
      | 18 r dot (rad/s2)
      | 19 fi dot (rad/s)
      | 20 theta dot (rad/s)
      | 21 psi dot (rad/s)
      | 22 xe dot (m/s)
      | 23 ye dot (m/s)
      | 24 ze dot (m/s)
      | 25 u dot (m/s2)
      | 26 v dot (m/s2)
      | 27 w dot (m/s2)
      | 28 pb/2v (rad)
      | 29 qc/v (rad)
      | 30 rb/v (rad)
      | 31 Ax (g)
      | 32 Ay (g)
      | 33 Az (g)
      | 34 ax (g)
      | 35 ay (g)
      | 36 az (g)
      | 37 delta elevators (rad)
      | 38 delta ailerons (rad)
      | 39 delta rudder (rad)
      | 40 delta stabs (rad)

== system RASCAL72_cl/RASCAL-72/ae/aero/Subsystem/Ma to Cn/Double click here for info 2 ==
  note: 01 v (m/s)
      | 02 alpha (rad)
      | 03 beta (rad)
      | 04 p (rad/s)
      | 05 q (rad/s)
      | 06 r  (rad/s)
      | 07 psi (rad)
      | 08 theta (rad)
      | 09 phi (rad)
      | 10 xe (m)
      | 11 ye (m)
      | 12 ze (m)
      | 13 v dot (m/s2)
      | 14 alpha dot (rad/s)
      | 15 beta dot (rad/s)
      | 16 p dot (rad/s2)
      | 17 q dot (rad/s2)
      | 18 r dot (rad/s2)
      | 19 fi dot (rad/s)
      | 20 theta dot (rad/s)
      | 21 psi dot (rad/s)
      | 22 xe dot (m/s)
      | 23 ye dot (m/s)
      | 24 ze dot (m/s)
      | 25 u dot (m/s2)
      | 26 v dot (m/s2)
      | 27 w dot (m/s2)
      | 28 pb/2v (rad)
      | 29 qc/v (rad)
      | 30 rb/v (rad)
      | 31 Ax (g)
      | 32 Ay (g)
      | 33 Az (g)
      | 34 ax (g)
      | 35 ay (g)
      | 36 az (g)
      | 37 delta elevators (rad)
      | 38 delta ailerons (rad)
      | 39 delta rudder (rad)
      | 40 delta stabs (rad)
